simulink model "ref_model2"  (R2022b)
settings: Solver=ode8  StartTime=0.0  StopTime=10.0  FixedStep=.01  RelTol=1e-3
values from neighbouring files (symbols this model uses):
  Ts = .05    (= 0.05)    [RunMeFirst.m]    (also in linsys1.m = 0.1)
settings Model: Creator=hp_desktop  LastModifiedBy=hp_desktop
settings ModelReferenceCC: UseModelRefSolver=on

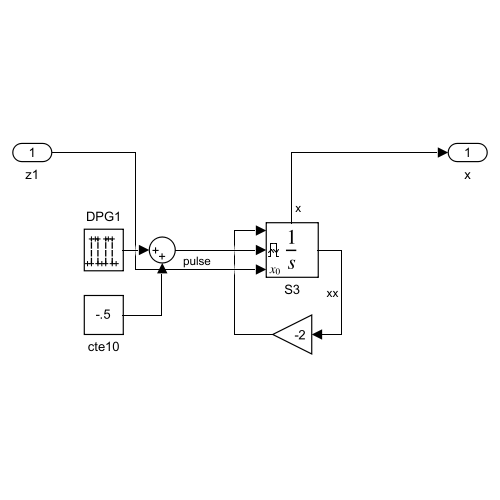
[thumbnail: Simulink's stored preview of the top-level diagram]
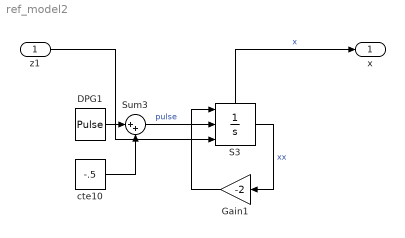
== system ref_model2 ==
  z1 : Inport
  DPG1 : DiscretePulseGenerator  SampleTime=Ts
  Gain1 : Gain  Gain=-2
  S3 : Integrator  ExternalReset=either  InitialConditionSource=external  ShowStatePort=on
  Sum3 : Sum  Inputs=|++
  cte10 : Constant  Value=-.5
  x : Outport
  wires:
  cte10/1 -> Sum3/2
  Sum3/1 -> S3/2  "pulse"
  Gain1/1 -> S3/1
  S3/State -> x/1  "x"
  z1/1 -> S3/3
  DPG1/1 -> Sum3/1
  S3/1 -> Gain1/1  "xx"
